simulink model "sistem_ordin_I_cu_timp_mort"  (R2023b)
settings: Solver=VariableStepAuto  StartTime=0.0  StopTime=30  MaxStep=1e-3  RelTol=1e-3
values from neighbouring files (symbols this model uses):
  b = 0.2    [sns_proiect_Ceoca_Ovidiu.m]
  den = [T 1]    [sns_proiect_Ceoca_Ovidiu.m]
  h1 = T/10    (= 0.2)    [sns_proiect_Ceoca_Ovidiu.m]
  Kp = 0.45*Ku    (= 0.450881601519)    [sns_proiect_Ceoca_Ovidiu.m]
  num = [1]    [sns_proiect_Ceoca_Ovidiu.m]
  taum = 1    [sns_proiect_Ceoca_Ovidiu.m]
  Ti = 0.8*Tosc    (= 8)    [sns_proiect_Ceoca_Ovidiu.m]
  Tt1 = 0.5    [sns_proiect_Ceoca_Ovidiu.m]
settings Model: Creator=ovidiuceoca  LastModifiedBy=ovidiuceoca

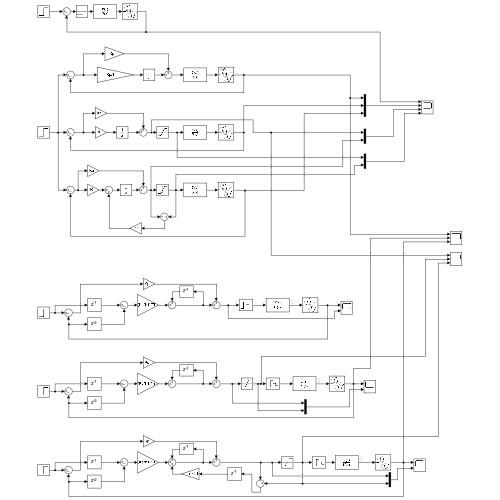
[thumbnail: Simulink's stored preview of the top-level diagram]
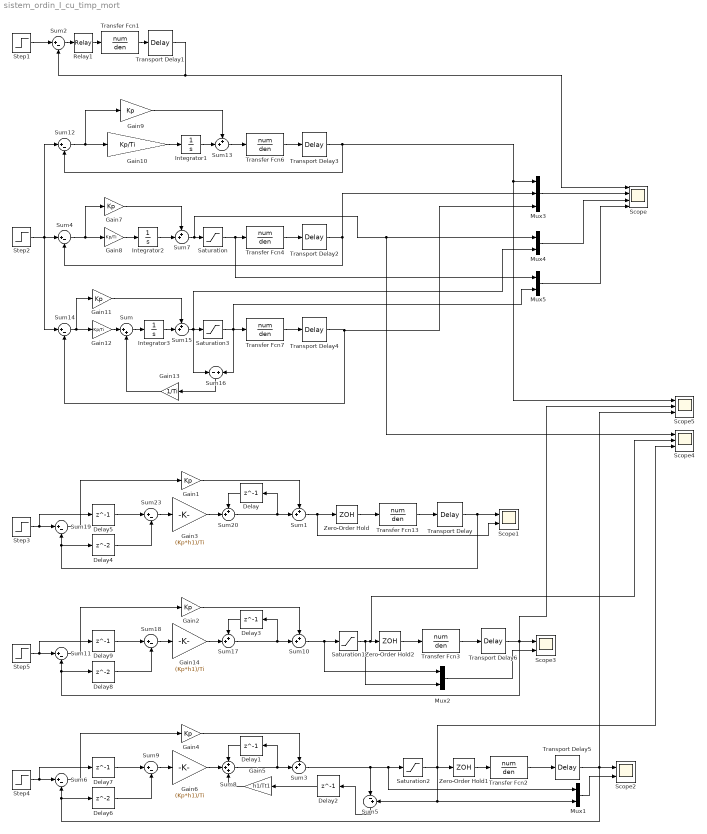
== system sistem_ordin_I_cu_timp_mort ==
  Delay{,1..3,5,7,9} (7 alike) : Delay  DelayLength=1  SampleTime=h1
  Delay4 : Delay  SampleTime=h1
  Delay6 : Delay  SampleTime=h1
  Delay8 : Delay  SampleTime=h1
  Gain{1..2,4,7,9,11} (6 alike) : Gain  Gain=Kp
  Gain10 : Gain  Gain=Kp/Ti
  Gain12 : Gain  Gain=Kp/Ti
  Gain13 : Gain  Gain=1/Ti
  Gain14 : Gain  Gain=(Kp*h1)/Ti
  Gain3 : Gain  Gain=(Kp*h1)/Ti
  Gain5 : Gain  Gain=h1/Tt1
  Gain6 : Gain  Gain=(Kp*h1)/Ti
  Gain8 : Gain  Gain=Kp/Ti
  Integrator1 : Integrator
  Integrator2 : Integrator
  Integrator3 : Integrator
  Mux{1..2,4..5} (4 alike) : Mux  Inputs=2
  Mux3 : Mux  Inputs=3
  Relay1 : Relay  OnSwitchValue=0  OffSwitchValue=0  OnOutputValue=b  OffOutputValue=-b
  Saturation : Saturate  UpperLimit=1.5  LowerLimit=-1.2
  Saturation1 : Saturate  UpperLimit=1.5  LowerLimit=-1.5
  Saturation2 : Saturate  UpperLimit=1.5  LowerLimit=-1.5
  Saturation3 : Saturate  UpperLimit=1.5  LowerLimit=-1.2
  Scope : Scope  NumInputPorts=4
  Scope1 : Scope  NumInputPorts=2
  Scope2 : Scope  NumInputPorts=2
  Scope3 : Scope  NumInputPorts=2
  Scope4 : Scope  NumInputPorts=3
  Scope5 : Scope  NumInputPorts=3
  Step1 : Step  Time=0  After=0.5  SampleTime=0
  Step{2..5} (4 alike) : Step  Time=0  SampleTime=0
  Sum : Sum  Inputs=|++
  Sum{1,3,7,10,13,15,17,20} (8 alike) : Sum  Inputs=++|
  Sum{2,4,6,9,11..12,14,18..19,23} (10 alike) : Sum  Inputs=|+-
  Sum16 : Sum  Inputs=-|+
  Sum5 : Sum  Inputs=|-+
  Sum8 : Sum  Inputs=+++
  Transfer Fcn{1..4,6..7,13} (7 alike) : TransferFcn  Numerator=num  Denominator=den
  Transport Delay{,1..6} (7 alike) : TransportDelay  DelayTime=taum
  Zero-Order Hold : ZeroOrderHold  SampleTime=h1
  Zero-Order Hold1 : ZeroOrderHold  SampleTime=h1
  Zero-Order Hold2 : ZeroOrderHold  SampleTime=h1
  wires:
  Integrator2/1 -> Sum7/2
  Gain8/1 -> Integrator2/1
  Gain7/1 -> Sum7/1
  Sum7/1 -> Scope4/1, Mux4/1, Saturation/1
  Sum4/1 -> Gain8/1, Gain7/1
  Transport Delay2/1 -> Sum4/2, Mux3/2
  Transfer Fcn4/1 -> Transport Delay2/1
  Saturation/1 -> Mux5/1, Transfer Fcn4/1
  Relay1/1 -> Transfer Fcn1/1
  Transport Delay1/1 -> Scope/1, Sum2/2
  Transfer Fcn1/1 -> Transport Delay1/1
  Sum2/1 -> Relay1/1
  Step1/1 -> Sum2/1
  Transfer Fcn6/1 -> Transport Delay3/1
  Gain9/1 -> Sum13/1
  Sum13/1 -> Transfer Fcn6/1
  Integrator1/1 -> Sum13/2
  Gain10/1 -> Integrator1/1
  Sum12/1 -> Gain9/1, Gain10/1
  Transport Delay3/1 -> Sum12/2, Mux3/1, Scope5/1
  Transfer Fcn7/1 -> Transport Delay4/1
  Gain11/1 -> Sum15/1
  Integrator3/1 -> Sum15/2
  Sum14/1 -> Gain12/1, Gain11/1
  Transport Delay4/1 -> Mux3/3, Sum14/2
  Saturation3/1 -> Mux5/2, Sum16/2, Transfer Fcn7/1
  Sum15/1 -> Mux4/2, Sum16/1, Saturation3/1
  Gain13/1 -> Sum/2
  Sum16/1 -> Gain13/1
  Gain12/1 -> Sum/1
  Sum/1 -> Integrator3/1
  Mux3/1 -> Scope/2
  Mux4/1 -> Scope/3
  Mux5/1 -> Scope/4
  Step2/1 -> Sum14/1, Sum12/1, Sum4/1
  Delay4/1 -> Sum23/2
  Zero-Order Hold/1 -> Transfer Fcn13/1
  Sum19/1 -> Gain1/1
  Delay5/1 -> Sum23/1
  Transfer Fcn13/1 -> Transport Delay/1
  Sum20/1 -> Sum1/2, Delay/1
  Delay/1 -> Sum20/1
  Gain1/1 -> Sum1/1
  Transport Delay/1 -> Scope1/1, Sum19/2, Delay4/1
  Sum23/1 -> Gain3/1
  Gain3/1 -> Sum20/2
  Step3/1 -> Delay5/1, Sum19/1
  Sum1/1 -> Scope1/2, Zero-Order Hold/1
  Delay7/1 -> Sum9/1
  Sum5/1 -> Delay2/1
  Sum3/1 -> Mux1/1, Saturation2/1, Sum5/1
  Transfer Fcn2/1 -> Transport Delay5/1
  Delay2/1 -> Gain5/1
  Sum8/1 -> Sum3/2, Delay1/1
  Saturation2/1 -> Mux1/2, Sum5/2, Scope4/3, Zero-Order Hold1/1
  Delay6/1 -> Sum9/2
  Gain4/1 -> Sum3/1
  Gain5/1 -> Sum8/3
  Delay1/1 -> Sum8/1
  Zero-Order Hold1/1 -> Transfer Fcn2/1
  Sum6/1 -> Gain4/1
  Transport Delay5/1 -> Scope5/3, Scope2/1, Sum6/2, Delay6/1
  Gain6/1 -> Sum8/2
  Sum9/1 -> Gain6/1
  Step4/1 -> Delay7/1, Sum6/1
  Mux1/1 -> Scope2/2
  Sum10/1 -> Mux2/1, Saturation1/1
  Step5/1 -> Sum11/1, Delay9/1
  Gain14/1 -> Sum17/2
  Sum18/1 -> Gain14/1
  Transport Delay6/1 -> Scope5/2, Delay8/1, Sum11/2, Scope3/1
  Gain2/1 -> Sum10/1
  Delay3/1 -> Sum17/1
  Sum17/1 -> Delay3/1, Sum10/2
  Transfer Fcn3/1 -> Transport Delay6/1
  Delay9/1 -> Sum18/1
  Sum11/1 -> Gain2/1
  Zero-Order Hold2/1 -> Transfer Fcn3/1
  Delay8/1 -> Sum18/2
  Saturation1/1 -> Scope4/2, Zero-Order Hold2/1, Mux2/2
  Mux2/1 -> Scope3/2
